simulink model "Simulink_PLC_coder_example_LAB_10"  (R2021b)
settings: Solver=FixedStepDiscrete  StartTime=0.0  StopTime=10  FixedStep=0.01  RelTol=1e-3
undefined symbols (not defined in the file): DiscIntNeverNeededParam
settings Model: Creator=Jan Størbu  LastModifiedBy=danielh
settings SolverCC: AlgebraicLoopSolver=TrustRegion
settings DataIOCC: ReturnWorkspaceOutputs=off
settings DebuggingCC: BusObjectLabelMismatch=error  SFMachineParentedDataDiag=warning  ArithmeticOperatorsInVariantConditions=warning
settings SFSimCC: SimUseLocalCustomCode=off  CustomCodeUndefinedFunction=UseInterfaceOnly
settings RTWCC: RTWUseLocalCustomCode=off
settings ConfigComp: PLC_TargetIDE=plcopen  PLC_MultiTBSigbuilderTimeRange=off  PLC_ReuseMLFcnVariable=on  PLC_InlineEnumCastFunction=off  PLC_GenerateReport=off  PLC_LaunchReport=off

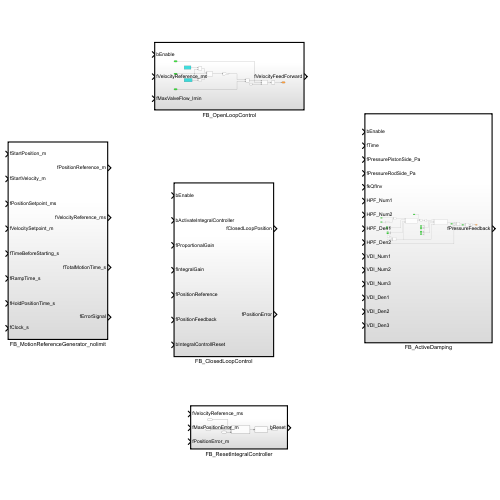
[thumbnail: Simulink's stored preview of the top-level diagram]
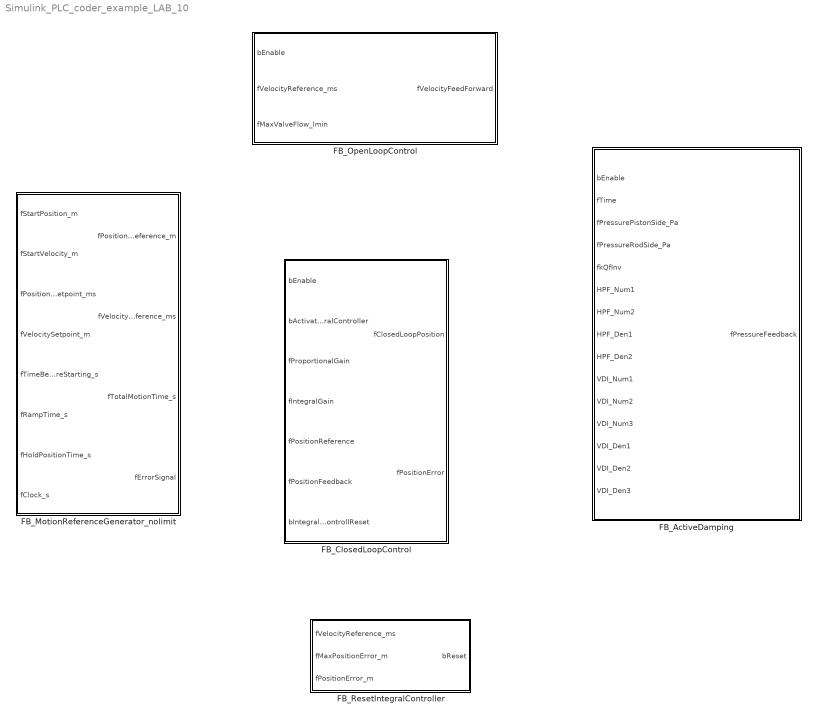
== system Simulink_PLC_coder_example_LAB_10 ==
  FB_ActiveDamping : Subsystem  TreatAsAtomicUnit=on
  FB_ClosedLoopControl : Subsystem  TreatAsAtomicUnit=on
  FB_MotionReferenceGenerator_nolimit : Subsystem  TreatAsAtomicUnit=on  VariantControl=Ramp_Profile
  FB_OpenLoopControl : Subsystem  TreatAsAtomicUnit=on
  FB_ResetIntegralController : Subsystem  TreatAsAtomicUnit=on

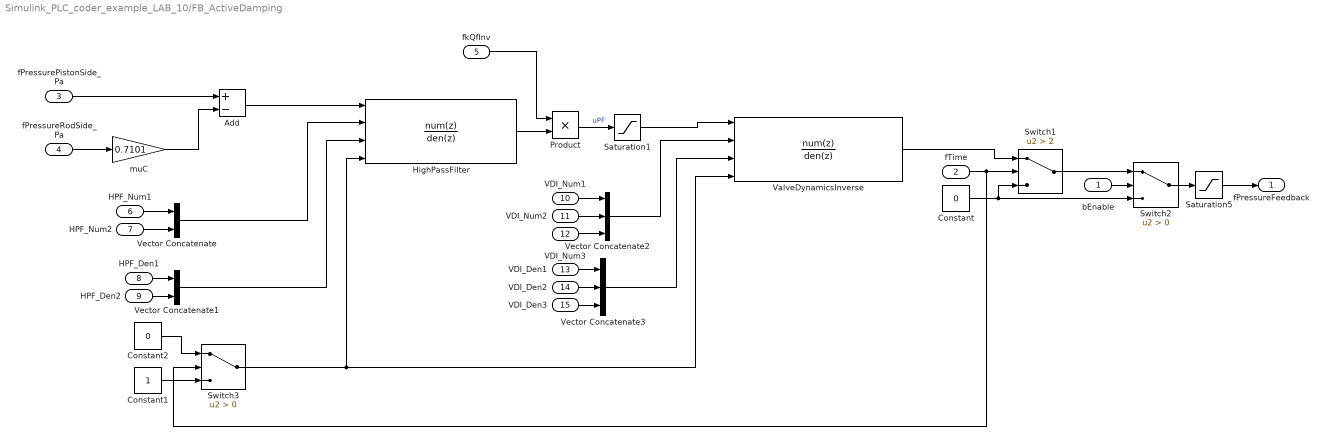
== system Simulink_PLC_coder_example_LAB_10/FB_ActiveDamping ==
  bEnable : Inport  OutDataTypeStr=boolean
  fTime : Inport  Port=2
  fPressurePistonSide_Pa : Inport  Port=3
  fPressureRodSide_Pa : Inport  Port=4
  fkQfInv : Inport  Port=5
  HPF_Num1 : Inport  Port=6
  HPF_Num2 : Inport  Port=7
  HPF_Den1 : Inport  Port=8
  HPF_Den2 : Inport  Port=9
  VDI_Num1 : Inport  Port=10
  VDI_Num2 : Inport  Port=11
  VDI_Num3 : Inport  Port=12
  VDI_Den1 : Inport  Port=13
  VDI_Den2 : Inport  Port=14
  VDI_Den3 : Inport  Port=15
  Add : Sum  Inputs=+-
  Constant : Constant  Value=0
  Constant1 : Constant
  Constant2 : Constant  Value=0
  HighPassFilter : DiscreteTransferFcn  NumeratorSource=Input port  Numerator=[3.786e-11 -3.786e-11]  DenominatorSource=Input port  Denominator=[1 -0.9954]  ExternalReset=Level hold  a0EqualsOne=on
      settings: InputPortMap=u0,p1,p3,r7
  Product : Product
  Saturation1 : Saturate  UpperLimit=1  LowerLimit=-1
  Saturation5 : Saturate  UpperLimit=1  LowerLimit=-1
  Switch1 : Switch  Criteria=u2 > Threshold  Threshold=2
  Switch2 : Switch  Criteria=u2 > Threshold
  Switch3 : Switch  Criteria=u2 > Threshold
  ValveDynamicsInverse : DiscreteTransferFcn  NumeratorSource=Input port  Numerator=[25 -48.83 23.85]  DenominatorSource=Input port  Denominator=[1 -1.721 0.7408]  ExternalReset=Level hold  a0EqualsOne=on
      settings: InputPortMap=u0,p1,p3,r7
  Vector Concatenate : Concatenate
  Vector Concatenate1 : Concatenate
  Vector Concatenate2 : Concatenate  NumInputs=3
  Vector Concatenate3 : Concatenate  NumInputs=3
  muC : Gain  Gain=0.7101
  fPressureFeedback : Outport  VectorParamsAs1DForOutWhenUnconnected=off
  wires:
  Add/1 -> HighPassFilter/1
  fPressurePistonSide_Pa/1 -> Add/1
  HighPassFilter/1 -> Product/2
  Constant/1 -> Switch1/3, Switch2/3
  fPressureRodSide_Pa/1 -> muC/1
  Switch2/1 -> Saturation5/1
  Switch1/1 -> Switch2/1
  bEnable/1 -> Switch2/2
  Saturation5/1 -> fPressureFeedback/1
  Vector Concatenate2/1 -> ValveDynamicsInverse/2
  Vector Concatenate3/1 -> ValveDynamicsInverse/3
  VDI_Den1/1 -> Vector Concatenate3/1
  VDI_Den2/1 -> Vector Concatenate3/2
  VDI_Den3/1 -> Vector Concatenate3/3
  ValveDynamicsInverse/1 -> Switch1/1
  fkQfInv/1 -> Product/1
  muC/1 -> Add/2
  VDI_Num1/1 -> Vector Concatenate2/1
  VDI_Num2/1 -> Vector Concatenate2/2
  VDI_Num3/1 -> Vector Concatenate2/3
  Saturation1/1 -> ValveDynamicsInverse/1
  Product/1 -> Saturation1/1  "uPF"
  fTime/1 -> Switch3/2, Switch1/2
  HPF_Num2/1 -> Vector Concatenate/2
  Vector Concatenate/1 -> HighPassFilter/2
  HPF_Num1/1 -> Vector Concatenate/1
  Vector Concatenate1/1 -> HighPassFilter/3
  HPF_Den2/1 -> Vector Concatenate1/2
  HPF_Den1/1 -> Vector Concatenate1/1
  Switch3/1 -> ValveDynamicsInverse/4, HighPassFilter/4
  Constant1/1 -> Switch3/3
  Constant2/1 -> Switch3/1

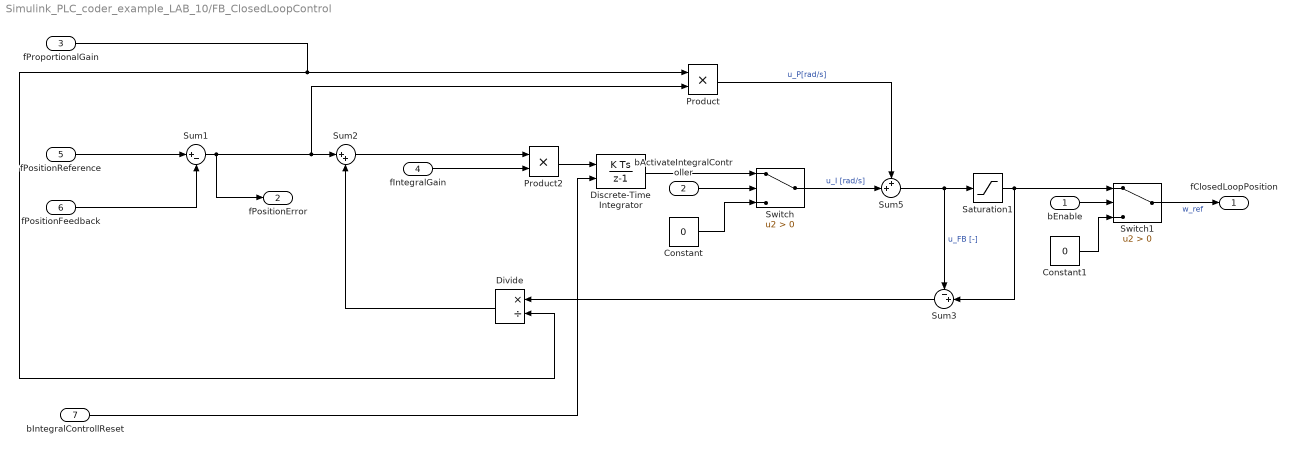
== system Simulink_PLC_coder_example_LAB_10/FB_ClosedLoopControl ==
  bEnable : Inport  OutDataTypeStr=boolean
  bActivateIntegralController : Inport  Port=2  OutDataTypeStr=boolean
  fProportionalGain : Inport  Port=3
  fIntegralGain : Inport  Port=4
  fPositionReference : Inport  Port=5
  fPositionFeedback : Inport  Port=6
  bIntegralControllReset : Inport  Port=7  OutDataTypeStr=boolean
  Constant : Constant  Value=0
  Constant1 : Constant  Value=0
  Discrete-Time Integrator : DiscreteIntegrator  ExternalReset=sampled level  SampleTime=-1  LimitOutput=on  UpperSaturationLimit=1  LowerSaturationLimit=-1  ICPrevOutput=DiscIntNeverNeededParam  ICPrevScaledInput=DiscIntNeverNeededParam
  Divide : Product  Inputs=*/
  Product : Product
  Product2 : Product
  Saturation1 : Saturate  UpperLimit=1  LowerLimit=-1
  Sum1 : Sum  Inputs=|+-
  Sum2 : Sum  Inputs=|++
  Sum3 : Sum  Inputs=-+|
  Sum5 : Sum  Inputs=++|
  Switch : Switch  Criteria=u2 > Threshold
  Switch1 : Switch  Criteria=u2 > Threshold
  fClosedLoopPosition : Outport  VectorParamsAs1DForOutWhenUnconnected=off
  fPositionError : Outport  Port=2  VectorParamsAs1DForOutWhenUnconnected=off
  wires:
  fPositionFeedback/1 -> Sum1/2
  Sum2/1 -> Product2/1
  Divide/1 -> Sum2/2
  fProportionalGain/1 -> Product/1, Divide/2
  fIntegralGain/1 -> Product2/2
  bActivateIntegralController/1 -> Switch/2
  Constant/1 -> Switch/3
  fPositionReference/1 -> Sum1/1
  Sum5/1 -> Sum3/1, Saturation1/1  "u_FB [-]"
  Sum3/1 -> Divide/1
  Switch1/1 -> fClosedLoopPosition/1  "w_ref"
  Constant1/1 -> Switch1/3
  bEnable/1 -> Switch1/2
  Saturation1/1 -> Switch1/1, Sum3/2
  Product/1 -> Sum5/1  "u_P[rad/s]"
  Switch/1 -> Sum5/2  "u_I [rad/s]"
  Product2/1 -> Discrete-Time Integrator/1
  bIntegralControllReset/1 -> Discrete-Time Integrator/2
  Discrete-Time Integrator/1 -> Switch/1
  Sum1/1 -> fPositionError/1, Product/2, Sum2/1

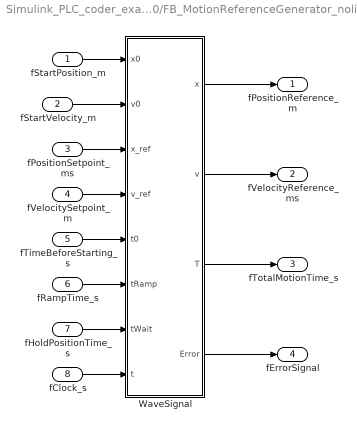
== system Simulink_PLC_coder_example_LAB_10/FB_MotionReferenceGenerator_nolimit ==
  fStartPosition_m : Inport
  fStartVelocity_m : Inport  Port=2
  fPositionSetpoint_ms : Inport  Port=3
  fVelocitySetpoint_m : Inport  Port=4
  fTimeBeforeStarting_s : Inport  Port=5
  fRampTime_s : Inport  Port=6
  fHoldPositionTime_s : Inport  Port=7
  fClock_s : Inport  Port=8
  WaveSignal : MATLAB Function  TreatAsAtomicUnit=on
  fPositionReference_m : Outport  VectorParamsAs1DForOutWhenUnconnected=off
  fVelocityReference_ms : Outport  Port=2  VectorParamsAs1DForOutWhenUnconnected=off
  fTotalMotionTime_s : Outport  Port=3  VectorParamsAs1DForOutWhenUnconnected=off
  fErrorSignal : Outport  Port=4  VectorParamsAs1DForOutWhenUnconnected=off
  wires:
  fClock_s/1 -> WaveSignal/8(t)
  fStartVelocity_m/1 -> WaveSignal/2(v0)
  fTimeBeforeStarting_s/1 -> WaveSignal/5(t0)
  fPositionSetpoint_ms/1 -> WaveSignal/3(x_ref)
  fHoldPositionTime_s/1 -> WaveSignal/7(tWait)
  fVelocitySetpoint_m/1 -> WaveSignal/4(v_ref)
  WaveSignal/3(T) -> fTotalMotionTime_s/1
  fStartPosition_m/1 -> WaveSignal/1(x0)
  fRampTime_s/1 -> WaveSignal/6(tRamp)
  WaveSignal/4(Error) -> fErrorSignal/1
  WaveSignal/1(x) -> fPositionReference_m/1
  WaveSignal/2(v) -> fVelocityReference_ms/1

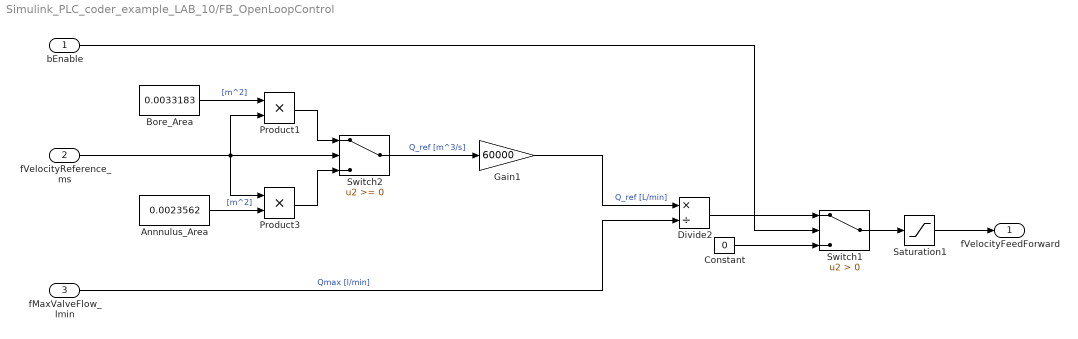
== system Simulink_PLC_coder_example_LAB_10/FB_OpenLoopControl ==
  bEnable : Inport  OutDataTypeStr=boolean
  fVelocityReference_ms : Inport  Port=2
  fMaxValveFlow_lmin : Inport  Port=3
  Annnulus_Area : Constant  Value=0.0023562
  Bore_Area : Constant  Value=0.0033183
  Constant : Constant  Value=0
  Divide2 : Product  Inputs=*/
  Gain1 : Gain  Gain=60000
  Product1 : Product
  Product3 : Product
  Saturation1 : Saturate  UpperLimit=1  LowerLimit=-1
  Switch1 : Switch  Criteria=u2 > Threshold
  Switch2 : Switch
  fVelocityFeedForward : Outport  VectorParamsAs1DForOutWhenUnconnected=off
  wires:
  Annnulus_Area/1 -> Product3/2  "[m^2]"
  Switch2/1 -> Gain1/1  "Q_ref [m^3/s]"
  Product1/1 -> Switch2/1
  fVelocityReference_ms/1 -> Product3/1, Product1/2, Switch2/2
  fMaxValveFlow_lmin/1 -> Divide2/2  "Qmax [l/min]"
  Bore_Area/1 -> Product1/1  "[m^2]"
  Gain1/1 -> Divide2/1  "Q_ref [L/min]"
  Product3/1 -> Switch2/3
  Constant/1 -> Switch1/3
  Divide2/1 -> Switch1/1
  bEnable/1 -> Switch1/2
  Switch1/1 -> Saturation1/1
  Saturation1/1 -> fVelocityFeedForward/1

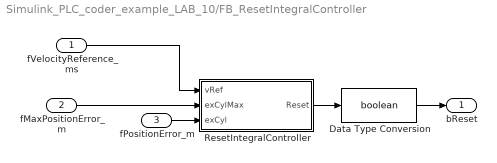
== system Simulink_PLC_coder_example_LAB_10/FB_ResetIntegralController ==
  fVelocityReference_ms : Inport
  fMaxPositionError_m : Inport  Port=2
  fPositionError_m : Inport  Port=3
  Data Type Conversion : DataTypeConversion  OutDataTypeStr=boolean
  ResetIntegralController : MATLAB Function  TreatAsAtomicUnit=on
  bReset : Outport  OutDataTypeStr=boolean
  wires:
  fMaxPositionError_m/1 -> ResetIntegralController/2(exCylMax)
  fVelocityReference_ms/1 -> ResetIntegralController/1(vRef)
  ResetIntegralController/1(Reset) -> Data Type Conversion/1
  fPositionError_m/1 -> ResetIntegralController/3(exCyl)
  Data Type Conversion/1 -> bReset/1

== matlab function Simulink_PLC_coder_example_LAB_10/FB_MotionReferenceGenerator_nolimit/WaveSignal ==
  data: x0 input; v0 input; x_ref input; x output; v_ref input; t0 input; tRamp input; tWait input; v output; t input; T output; Error output double
function [x,v,T, Error] = fcn(x0,v0, x_ref,v_ref,t0,tRamp,tWait,t)
x_SP = x_ref - x0;
vs=v_ref;
slopeExt=v0-vs;
slopeRetr=-vs-v0;

as = vs/tRamp;
s_acc=(vs^2-v0^2)/as;

tHold=(x_SP-s_acc)/vs;

if tHold < 0 
Error = 1;
else 
Error = 0;
end

t1=tRamp;
t2=tHold; 
t3=tRamp;
t4=tWait;
t5=t1;
t6=t2;
t7=t3;

x = x0;
x1 = x0 + v0*((t0+t1)-t0)-(slopeExt/t1)*((t0+t1)-t0)^2/2;
x2 = x1 + vs*((t0+t1+t2)-(t0+t1)); 
x4 = x_ref - v0*((t0+t1+t2+t3+t4+t5)-(t0+t1+t2+t3+t4))+(slopeRetr/t5)*((t0+t1+t2+t3+t4+t5)-(t0+t1+t2+t3+t4))^2/2; 
x5 = x4-vs*((t0+t1+t2+t3+t4+t5+t6)-(t0+t1+t2+t3+t4+t5));  

if Error == 1
x = x0;
v = v0; 
elseif t>=0 && t<t0
x = x0; 
v = v0;
elseif t>=t0 && t<(t0+t1)
x = x0 + v0*(t-t0)-(slopeExt/t1)*(t-t0)^2/2;
v = v0-(slopeExt/t1)*(t-t0);  
elseif t>=(t0+t1) && t<(t0+t1+t2)
x = x1 + vs*(t-(t0+t1)); 
v = vs; 
elseif t>=(t0+t1+t2) && t<(t0+t1+t2+t3)
x = x2+vs*(t-(t0+t1+t2))+(slopeExt/t3)*(t-(t0+t1+t2))^2/2; 
v = vs+(slopeExt/t3)*(t-(t0+t1+t2));   
elseif t>=(t0+t1+t2+t3) && t<(t0+t1+t2+t3+t4)
x = x_ref;
v = v0;  
elseif t>=(t0+t1+t2+t3+t4) && t<(t0+t1+t2+t3+t4+t5)
x = x_ref - v0*(t-(t0+t1+t2+t3+t4))+(slopeRetr/t5)*(t-(t0+t1+t2+t3+t4))^2/2; 
v = v0+(slopeRetr/t5)*(t-(t0+t1+t2+t3+t4));     
elseif t>=(t0+t1+t2+t3+t4+t5) && t<(t0+t1+t2+t3+t4+t5+t6)
x = x4-vs*(t-(t0+t1+t2+t3+t4+t5));   
v = -vs;    
elseif t>=(t0+t1+t2+t3+t4+t5+t6) && t<(t0+t1+t2+t3+t4+t5+t6+t7)
x = x5-vs*(t-(t0+t1+t2+t3+t4+t5+t6))-(slopeRetr/t3)*(t-(t0+t1+t2+t3+t4+t5+t6))^2/2;    
v = -vs-(slopeRetr/t3)*(t-(t0+t1+t2+t3+t4+t5+t6));     
else 
x = x0;
v = v0; 
end

T = t0+t1+t2+t3+t4+t5+t6+t7;

== matlab function Simulink_PLC_coder_example_LAB_10/FB_ResetIntegralController/ResetIntegralController ==
  data: vRef input; exCylMax input; Reset output; exCyl input
function Reset = fcn(vRef, exCylMax, exCyl)

if abs(vRef) > 0 || abs(exCyl) > exCylMax
Reset = 0;
else 
Reset = 1;
end
